simulink model "model"  (R2020b)
settings: Solver=ode3  StartTime=0.0  StopTime=stop_time  FixedStep=Ts  RelTol=1e-3
values from neighbouring files (symbols this model uses):
  L = u(6)    [f.m]    (also in main.m = 1)
  R = u(5)    [f.m]    (also in main.m = 0.95)
  x_0 = [0; 0; 0; 0]    [main.m]
settings Model: Creator=fanyang  LastModifiedBy=fanyang

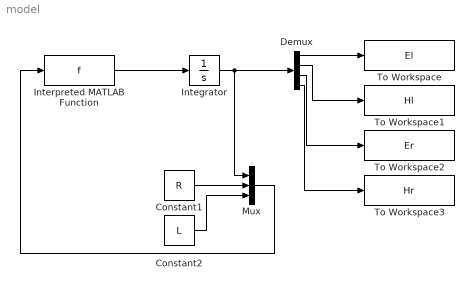
== system model ==
  Constant1 : Constant  Value=R
  Constant2 : Constant  Value=L
  Demux : Demux
  Integrator : Integrator  InitialCondition=x_0
  Interpreted MATLAB Function : MATLABFcn  MATLABFcn=f  OutputDimensions=4
  Mux : Mux  Inputs=3
  To Workspace : ToWorkspace  VariableName=El  SaveFormat=Timeseries  SampleTime=-1
  To Workspace1 : ToWorkspace  VariableName=Hl  SaveFormat=Timeseries  SampleTime=-1
  To Workspace2 : ToWorkspace  VariableName=Er  SaveFormat=Timeseries  SampleTime=-1
  To Workspace3 : ToWorkspace  VariableName=Hr  SaveFormat=Timeseries  SampleTime=-1
  wires:
  Interpreted MATLAB Function/1 -> Integrator/1
  Integrator/1 -> Demux/1, Mux/1
  Mux/1 -> Interpreted MATLAB Function/1
  Constant1/1 -> Mux/2
  Constant2/1 -> Mux/3
  Demux/1 -> To Workspace/1
  Demux/2 -> To Workspace1/1
  Demux/3 -> To Workspace2/1
  Demux/4 -> To Workspace3/1
